simulink model "SEND_model"  (Simulink 6.4)
settings: Solver=FixedStepDiscrete  StartTime=0.0  StopTime=inf  FixedStep=0.001  RelTol=1e-3
libraries: RT x1
settings Model: LastModifiedBy=Maggia

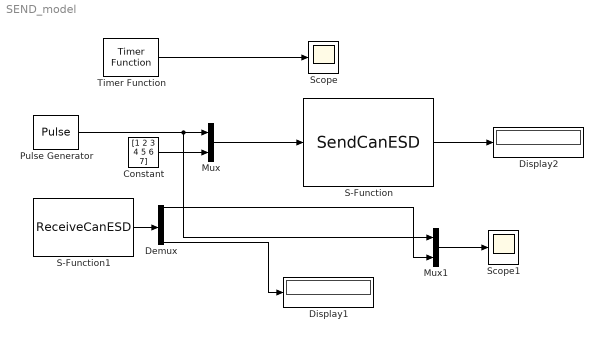
== system SEND_model ==
  Constant : Constant  Value=[1 2 3 4 5 6 7]  OutDataType=sfix(16)  ConRadixGroup=Use specified scaling  OutScaling=2^0  SampleTime=inf  FramePeriod=inf
  Demux : Demux  Outputs=8
  Display1 : Display
  Display2 : Display
  Mux : Mux  Inputs=2
  Mux1 : Mux  Inputs=2
  Pulse Generator : DiscretePulseGenerator  PulseType=Time based  Period=0.01  PulseWidth=50
  S-Function : S-Function  FunctionName=SendCanESD  Parameters=(baudrate-1),msgid,length  mask{baudrate=1000 Kbits/s, msgid=1823, length=8}
      mask prompts: msgid "Message ID"; length "Message Length"
      mask StyleString: popup(1000 Kbits/s|500  Kbits/s),edit,edit
      mask Display:
      | fprintf('SEND CAN\n')
      | fprintf('\nID %d',msgid);
      | port_label('input',1,'message');
      | color('red');port_label('output',1,'status');
  S-Function1 : S-Function  FunctionName=ReceiveCanESD  Parameters=msgID  mask{msgID=1200}
      mask prompts: msgID "Message ID"
  Scope : Scope
      settings: YMin=0  YMax=1200
  Scope1 : Scope
      settings: YMin=0  YMax=1
  Timer Function : RT/Timer Function  Priority=266597344  step=1  priority=HIGH  ThPriority=TIME CRITICAL
  wires:
  S-Function/1 -> Display2/1
  Mux/1 -> S-Function/1
  Pulse Generator/1 -> Mux/1, Mux1/1
  Constant/1 -> Mux/2
  Timer Function/1 -> Scope/1
  S-Function1/1 -> Demux/1
  Mux1/1 -> Scope1/1
  Demux/1 -> Mux1/2
  Demux/8 -> Display1/1
